simulink model "satellite"  (R2018a)
settings: Solver=ode23t  StartTime=0.0  StopTime=3600*24*2  FixedStep=1  RelTol=1e-6
libraries: simulink x1
settings Model: Creator=Martin  LastModifiedBy=Martin

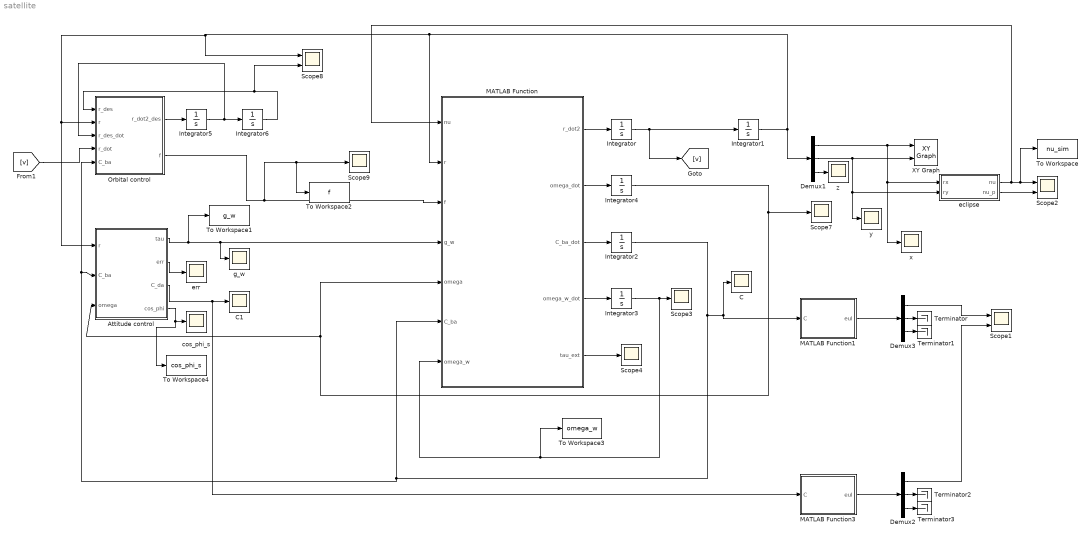
== system satellite ==
  Attitude control : MATLAB Function  TreatAsAtomicUnit=on
  C : Scope
  C1 : Scope
  Demux1 : Demux  Outputs=3
  Demux2 : Demux  Outputs=3
  Demux3 : Demux  Outputs=3
  Integrator : Integrator  InitialCondition=[0; 3.0690; 0]
  Integrator1 : Integrator  InitialCondition=[-42164 ; 0 ; 0]
  Integrator2 : Integrator  InitialCondition=eye(3)
  Integrator3 : Integrator  InitialCondition=[0; 0; 0]
  Integrator4 : Integrator  InitialCondition=[0;0;0]
  Integrator5 : Integrator  InitialCondition=[0; 3.0690; 0]
  Integrator6 : Integrator  InitialCondition=[-42164 ; 0 ; 0]
  MATLAB Function : MATLAB Function  TreatAsAtomicUnit=on
  MATLAB Function1 : MATLAB Function  TreatAsAtomicUnit=on
  MATLAB Function3 : MATLAB Function  TreatAsAtomicUnit=on
  Orbital control : MATLAB Function  TreatAsAtomicUnit=on
  Scope1 : Scope  NumInputPorts=2
  Scope2 : Scope  NumInputPorts=2
  Scope{3..4,7,9} (4 alike) : Scope
  Scope8 : Scope  NumInputPorts=2
  Terminator{,1..3} (4 alike) : Terminator
  To Workspace : ToWorkspace  VariableName=nu_sim  SaveFormat=Timeseries  SampleTime=-1
  To Workspace1 : ToWorkspace  VariableName=g_w  SaveFormat=Timeseries  SampleTime=-1
  To Workspace2 : ToWorkspace  VariableName=f  SaveFormat=Timeseries  SampleTime=-1
  To Workspace3 : ToWorkspace  VariableName=omega_w  SaveFormat=Timeseries  SampleTime=-1
  To Workspace4 : ToWorkspace  VariableName=cos_phi_s  SaveFormat=Timeseries  SampleTime=-1
  XY Graph : simulink/Sinks/XY Graph  xmin=-45000  xmax=45000  ymin=-45000  ymax=45000  st=-1
  "cos_phi_s " : Scope
  eclipse : MATLAB Function  TreatAsAtomicUnit=on
  err : Scope
  g_w : Scope
  x : Scope
  y : Scope
  z : Scope
  wires:
  MATLAB Function/1(r_dot2) -> Integrator/1
  Integrator/1 -> Integrator1/1, [v]
  Integrator1/1 -> Demux1/1, Scope8/1, Attitude control/1(r), Orbital control/2(r), MATLAB Function/2(r)
  MATLAB Function/2(omega_dot) -> Integrator4/1
  eclipse/1(nu) -> MATLAB Function/1(nu), To Workspace/1, Scope2/1
  Integrator4/1 -> Scope7/1, MATLAB Function/5(omega), Attitude control/3(omega)
  eclipse/2(nu_p) -> Scope2/2
  Demux1/1 -> x/1, eclipse/1(rx), XY Graph/1
  Demux1/2 -> y/1, eclipse/2(ry), XY Graph/2
  Demux1/3 -> z/1
  MATLAB Function/3(C_ba_dot) -> Integrator2/1
  Integrator2/1 -> MATLAB Function1/1(C), C/1, Orbital control/5(C_ba), Attitude control/2(C_ba), MATLAB Function/6(C_ba)
  Attitude control/2(err) -> err/1
  Attitude control/3(C_da) -> C1/1, MATLAB Function3/1(C)
  MATLAB Function1/1(eul) -> Demux3/1
  Attitude control/1(tau) -> MATLAB Function/4(g_w), g_w/1, To Workspace1/1
  MATLAB Function3/1(eul) -> Demux2/1
  Demux3/1 -> Scope1/1
  Demux2/1 -> Scope1/2
  MATLAB Function/4(omega_w_dot) -> Integrator3/1
  Integrator3/1 -> Scope3/1, To Workspace3/1, MATLAB Function/7(omega_w)
  MATLAB Function/5(tau_ext) -> Scope4/1
  Orbital control/1(r_dot2_des) -> Integrator5/1
  Integrator5/1 -> Integrator6/1, Orbital control/3(r_des_dot)
  Integrator6/1 -> Scope8/2, Orbital control/1(r_des)
  [v] -> Orbital control/4(r_dot)
  Demux3/2 -> Terminator/1
  Demux3/3 -> Terminator1/1
  Demux2/2 -> Terminator2/1
  Demux2/3 -> Terminator3/1
  Orbital control/2(f) -> To Workspace2/1, Scope9/1, MATLAB Function/3(f)
  Attitude control/4(cos_phi) -> To Workspace4/1, "cos_phi_s "/1

== matlab function satellite/eclipse ==
  data: rx input; nu output; ry input; nu_p output
function [nu,  nu_p] = fcn(rx, ry)
R_sun =  696e+3 ; 
R_earth = 6378.0 ;
AU = 149597870 ; 
r0 = 42164; 
r_sun_earth = [-AU ; 0]; 
r_sat_earth = [rx; ry]; 
chi = R_earth / (R_sun -R_earth)* norm(r_sun_earth); 
a_e = asin(R_earth/chi);
theta = r_sun_earth'*r_sat_earth / (norm(r_sun_earth)*norm(r_sat_earth));

% a = pi - acos (theta) ; 
% gamma = (2*chi*cos(a_e) - sqrt( (2*chi*cos(a_e))^2 - 4*(chi^2-r0^2) )) /2; 
% a_e2 = acos(  (gamma^2 - r0^2 - chi^2) /(-2*r0*chi)); 
% condition : abs(a) < a_e2 

s = [1; 0]; 
r_proj_earth = (s'*r_sat_earth)*s; 
delta = r_sat_earth - r_proj_earth;  
xi = (chi -  norm(r_proj_earth))*tan(a_e);

%% Umbra 
if (norm(delta) <= xi && (s'*r_sat_earth) > 0)
    nu_u = 0;  
else 
    nu_u = 1; 
end 

%% Penumbra 
chi_p = R_earth / (R_sun + R_earth)* norm(r_sun_earth); 
a_p = asin(R_earth/chi_p);
kappa = (chi_p + norm(r_proj_earth))*tan(a_p);

if (norm(delta) <= kappa && (s'*r_sat_earth) > 0)
    nu_p = (norm(delta)  -xi)/(kappa-xi);  
else 
    nu_p = 1; 
end 

nu = nu_u*nu_p;

== matlab function satellite/MATLAB Function ==
  data: nu input; r input; f input; g_w input; omega input; r_dot2 output; omega_dot output; C_ba input; C_ba_dot output; omega_w input; omega_w_dot output; tau_ext output
function [r_dot2, omega_dot, C_ba_dot, omega_w_dot , tau_ext]= fcn(nu, r, f, g_w, omega, C_ba, omega_w)
mu= 3.986004418e+14*1e-9; 
I=diag([1.1756e+04; 1.1756e+04; 5100]); 
I_w=22.5000; 
J=I +I_w;
m=3551; 
p = 4.5*10^(-6);
AU = 149597870 ; 
r_sun_earth = [-AU ; 0 ; 0];
A = 108; 
l_SA = 2.0*18.0 + 3; %length lever arm for solar force

% Orbital dynamics
F_s = p*A*(r+r_sun_earth)/norm(r+r_sun_earth)*nu; %solar radiation force
r_dot2 = -mu*r/norm(r)^3 + F_s + 1/m*C_ba'*f; % EOM update

% Attitude dynamics
r_b = C_ba * r; 
ratio_p = 161/85670; % ratio time in half penumbra vs orbit periode 
arc_p = 2*pi*norm(r)*ratio_p; % arc length of half penumbra section 
dec = l_SA / arc_p;
if (nu < 1) % only in penumbra 
tau_SA = [0 ; 0; sign(r(2))*norm(F_s)*l_SA^2/6*dec]; % solar torque
else 
tau_SA = [0 ; 0; 0];
end 
tau_grav= (3*mu/norm(r)^5)* cross(r_b) * J * r_b ; % gravity gradient
tau_ext = tau_SA + tau_grav; % external torques 
omega_dot = I^(-1)*( - cross(omega) *( J * omega + I_w*omega_w )   - g_w + tau_ext); % EOM update


% Wheel dynamics
 omega_w_dot  =  g_w/I_w - omega_dot ; % EOM update

% Rotational kinematics
C_ba_dot = - cross(omega)*C_ba; % EOM update

== matlab function satellite/Attitude control ==
  data: r input; C_ba input; omega input; tau output; err output; C_da output; cos_phi output
function [tau,err, C_da, cos_phi]= fcn(r, C_ba, omega)
% Tracking type
sw=1; % 1: earth pointing, other: sun pointing
% Gains
 k = 0.012/10;
 u_max = 3*1200e-3;
 w_max = u_max*(1-k);
 Kp = k*u_max/pi;
 AU = 149597870 ; 
 r_sun_earth = [-AU ; 0 ; 0];
 s = -(r + r_sun_earth)/norm(r + r_sun_earth); % unit vector pointing towards sun
 n_panel  = C_ba'*[1; 0; 0]; % solar panel normal 
 cos_phi = s'*n_panel; % cosine between solar panel normal and sun line of sight 
 
% Desired DCM (earth pointing)
if (sw==1)
r_d = r(1:end-1)/norm(r(1:end-1)); % (x,y)
x_a = [1;0]; y_a =[0;1]; % inertial basis vectors

C_da = [-r_d'*x_a   -r_d'*y_a    0;...
         r_d'*y_a   -r_d'*x_a    0;...
             0          0        1 ];
% Desired DCM (sun pointing)
else
x_a = [1;0;0]; y_a =[0;1;0]; % inertial basis vectors
s_y = [-s(2) ; s(1); 0];

C_da = [s'*x_a     s'*y_a      0;...
        s_y'*x_a   s_y'*y_a    0;...
             0          0      1 ];
end 
C_bd  = C_ba*C_da'; % error DCM

P = .5*(C_bd - C_bd'); % projection from SO(3) -> so(3) 

tau = Kp*vex(P)/sqrt(1+trace(C_bd))-sigma(omega, w_max); % control torque
tau = -tau; 
err = vex(P); % error metrics
end

function tau_d =sigma(u, w_max)
tau_d = max(-w_max,min(w_max, u)); 
end

== matlab function satellite/MATLAB Function1 ==
  data: C input; eul output
function eul= fcn(C)
% DCM to Euler
phi = atan2(C(1,2),C(1,1));
theta = asin(-C(1,3)); 
psi = atan2(C(2,3),C(3,3)); 
eul = [phi; theta; psi];

== matlab function satellite/MATLAB Function3 ==
  data: C input; eul output
function eul= fcn(C)
% DCM to Euler
phi = atan2(C(1,2),C(1,1));
theta = asin(-C(1,3)); 
psi = atan2(C(2,3),C(3,3)); 
eul = [phi; theta; psi];

== matlab function satellite/Orbital control ==
  data: r_des input; r_dot2_des output; r input; r_des_dot input; r_dot input; f output; C_ba input
function [r_dot2_des, f]   = fcn(r_des, r, r_des_dot, r_dot, C_ba)
mu= 3.986004418e+14*1e-9;
m=3551; 

kp=.1; 
kd=.1; 

f = m*C_ba*(kp*(r_des - r) + kd*(r_des_dot - r_dot)) ; 

r_dot2_des = -mu*r_des/norm(r_des)^3;
